simulink model "ctrl_custom"  (R2016b)
settings: Solver=ode4  StartTime=0.0  StopTime=500  FixedStep=0.01  RelTol=1e-3  EnableMultiTasking=on
libraries: simulink x2
(part 2 of 2)

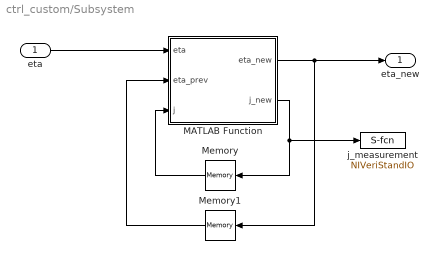
== system ctrl_custom/Subsystem ==
  eta : Inport
  MATLAB Function : MATLAB Function  TreatAsAtomicUnit=on
  Memory : Memory
  Memory1 : Memory  X0=[0;0;0]
  "j_measurement " : S-Function  Priority=1  FunctionName=NIVeriStandIO  Parameters=width dtype portnum stime stype btype  SFunctionDeploymentMode=off  EnableBusSupport=off  mask(NI VeriStand Outport){portnum=1, width=-1, stime=-1, dtype=auto, stype=auto, btype=0}
      mask prompts: portnum "Port number:"; width "Port dimensions (-1 for dynamically sized):"; stime "Sample time (-1 for inherited):"; dtype "Data type:"; stype "Signal type:"; btype "Block type:"
      mask help: Use this outport on any level of nested subsystems to allow NI VeriStand software to map signals to it.
      mask init:
      | NIVeriStandIO_init;
      settings: CopyFcn=NIVeriStand_MDL_functions('', 'IO_copy');  DeleteFcn=NIVeriStand_MDL_functions('', 'IO_delete');  MoveFcn=set_param(gcb, 'Mask', 'on');
      mask Callback portnum: NIVeriStand_MDL_functions('', 'IO_setportnum');
      mask TypeOptions dtype: auto | double | single | int8 | uint8 | int16 | uint16 | int32 | uint32 | boolean
      mask Callback dtype: NIVeriStand_MDL_functions('', 'IO_booleansignal');
      mask TypeOptions stype: auto | real | complex
      mask Display:
      | patch([-x x], [-y y], [.90980 .81960 .32156]);
      | plot([xrad -x x xrad], [yrad -y y yrad]);
      | fprintf('NI Out%d', portnum);
  eta_new : Outport
  wires:
  MATLAB Function/1(eta_new) -> Memory1/1, eta_new/1
  eta/1 -> MATLAB Function/1(eta)
  MATLAB Function/2(j_new) -> "j_measurement "/1, Memory/1
  Memory/1 -> MATLAB Function/3(j)
  Memory1/1 -> MATLAB Function/2(eta_prev)

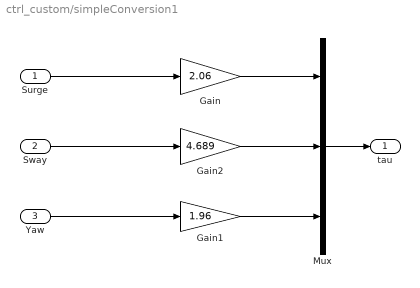
== system ctrl_custom/simpleConversion1 ==
  Surge : Inport
  Sway : Inport  Port=2
  Yaw : Inport  Port=3
  Gain : Gain  Gain=2.06
  Gain1 : Gain  Gain=1.96
  Gain2 : Gain  Gain=4.689
  Mux : Mux  Inputs=3
  "tau " : Outport
  wires:
  Yaw/1 -> Gain1/1
  Gain/1 -> Mux/1
  Mux/1 -> "tau "/1
  Surge/1 -> Gain/1
  Gain1/1 -> Mux/3
  Sway/1 -> Gain2/1
  Gain2/1 -> Mux/2

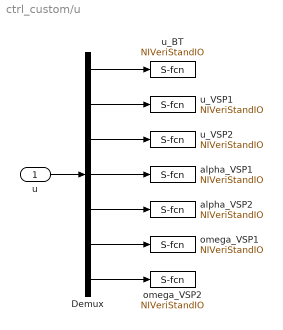
== system ctrl_custom/u ==
  u : Inport
  Demux : Demux  Outputs=7
  alpha_VSP1 : S-Function  Priority=4  FunctionName=NIVeriStandIO  Parameters=width dtype portnum stime stype btype  SFunctionDeploymentMode=off  EnableBusSupport=off  mask(NI VeriStand Outport){portnum=4, width=-1, stime=-1, dtype=auto, stype=auto, btype=0}
      mask prompts: portnum "Port number:"; width "Port dimensions (-1 for dynamically sized):"; stime "Sample time (-1 for inherited):"; dtype "Data type:"; stype "Signal type:"; btype "Block type:"
      mask help: Use this outport on any level of nested subsystems to allow NI VeriStand software to map signals to it.
      mask init:
      | NIVeriStandIO_init;
      settings: CopyFcn=NIVeriStand_MDL_functions('', 'IO_copy');  DeleteFcn=NIVeriStand_MDL_functions('', 'IO_delete');  MoveFcn=set_param(gcb, 'Mask', 'on');
      mask Callback portnum: NIVeriStand_MDL_functions('', 'IO_setportnum');
      mask TypeOptions dtype: auto | double | single | int8 | uint8 | int16 | uint16 | int32 | uint32 | boolean
      mask Callback dtype: NIVeriStand_MDL_functions('', 'IO_booleansignal');
      mask TypeOptions stype: auto | real | complex
      mask Display:
      | patch([-x x], [-y y], [.90980 .81960 .32156]);
      | plot([xrad -x x xrad], [yrad -y y yrad]);
      | fprintf('NI Out%d', portnum);
  alpha_VSP2 : S-Function  Priority=1  FunctionName=NIVeriStandIO  Parameters=width dtype portnum stime stype btype  SFunctionDeploymentMode=off  EnableBusSupport=off  mask(NI VeriStand Outport){portnum=1, width=-1, stime=-1, dtype=auto, stype=auto, btype=0}
      mask prompts: portnum "Port number:"; width "Port dimensions (-1 for dynamically sized):"; stime "Sample time (-1 for inherited):"; dtype "Data type:"; stype "Signal type:"; btype "Block type:"
      mask help: Use this outport on any level of nested subsystems to allow NI VeriStand software to map signals to it.
      mask init:
      | NIVeriStandIO_init;
      settings: CopyFcn=NIVeriStand_MDL_functions('', 'IO_copy');  DeleteFcn=NIVeriStand_MDL_functions('', 'IO_delete');  MoveFcn=set_param(gcb, 'Mask', 'on');
      mask Callback portnum: NIVeriStand_MDL_functions('', 'IO_setportnum');
      mask TypeOptions dtype: auto | double | single | int8 | uint8 | int16 | uint16 | int32 | uint32 | boolean
      mask Callback dtype: NIVeriStand_MDL_functions('', 'IO_booleansignal');
      mask TypeOptions stype: auto | real | complex
      mask Display:
      | patch([-x x], [-y y], [.90980 .81960 .32156]);
      | plot([xrad -x x xrad], [yrad -y y yrad]);
      | fprintf('NI Out%d', portnum);
  omega_VSP1 : S-Function  Priority=2  FunctionName=NIVeriStandIO  Parameters=width dtype portnum stime stype btype  SFunctionDeploymentMode=off  EnableBusSupport=off  mask(NI VeriStand Outport){portnum=2, width=-1, stime=-1, dtype=auto, stype=auto, btype=0}
      mask prompts: portnum "Port number:"; width "Port dimensions (-1 for dynamically sized):"; stime "Sample time (-1 for inherited):"; dtype "Data type:"; stype "Signal type:"; btype "Block type:"
      mask help: Use this outport on any level of nested subsystems to allow NI VeriStand software to map signals to it.
      mask init:
      | NIVeriStandIO_init;
      settings: CopyFcn=NIVeriStand_MDL_functions('', 'IO_copy');  DeleteFcn=NIVeriStand_MDL_functions('', 'IO_delete');  MoveFcn=set_param(gcb, 'Mask', 'on');
      mask Callback portnum: NIVeriStand_MDL_functions('', 'IO_setportnum');
      mask TypeOptions dtype: auto | double | single | int8 | uint8 | int16 | uint16 | int32 | uint32 | boolean
      mask Callback dtype: NIVeriStand_MDL_functions('', 'IO_booleansignal');
      mask TypeOptions stype: auto | real | complex
      mask Display:
      | patch([-x x], [-y y], [.90980 .81960 .32156]);
      | plot([xrad -x x xrad], [yrad -y y yrad]);
      | fprintf('NI Out%d', portnum);
  omega_VSP2 : S-Function  Priority=3  FunctionName=NIVeriStandIO  Parameters=width dtype portnum stime stype btype  SFunctionDeploymentMode=off  EnableBusSupport=off  mask(NI VeriStand Outport){portnum=3, width=-1, stime=-1, dtype=auto, stype=auto, btype=0}
      mask prompts: portnum "Port number:"; width "Port dimensions (-1 for dynamically sized):"; stime "Sample time (-1 for inherited):"; dtype "Data type:"; stype "Signal type:"; btype "Block type:"
      mask help: Use this outport on any level of nested subsystems to allow NI VeriStand software to map signals to it.
      mask init:
      | NIVeriStandIO_init;
      settings: CopyFcn=NIVeriStand_MDL_functions('', 'IO_copy');  DeleteFcn=NIVeriStand_MDL_functions('', 'IO_delete');  MoveFcn=set_param(gcb, 'Mask', 'on');
      mask Callback portnum: NIVeriStand_MDL_functions('', 'IO_setportnum');
      mask TypeOptions dtype: auto | double | single | int8 | uint8 | int16 | uint16 | int32 | uint32 | boolean
      mask Callback dtype: NIVeriStand_MDL_functions('', 'IO_booleansignal');
      mask TypeOptions stype: auto | real | complex
      mask Display:
      | patch([-x x], [-y y], [.90980 .81960 .32156]);
      | plot([xrad -x x xrad], [yrad -y y yrad]);
      | fprintf('NI Out%d', portnum);
  u_BT : S-Function  Priority=5  FunctionName=NIVeriStandIO  Parameters=width dtype portnum stime stype btype  SFunctionDeploymentMode=off  EnableBusSupport=off  mask(NI VeriStand Outport){portnum=5, width=-1, stime=-1, dtype=auto, stype=auto, btype=0}
      mask prompts: portnum "Port number:"; width "Port dimensions (-1 for dynamically sized):"; stime "Sample time (-1 for inherited):"; dtype "Data type:"; stype "Signal type:"; btype "Block type:"
      mask help: Use this outport on any level of nested subsystems to allow NI VeriStand software to map signals to it.
      mask init:
      | NIVeriStandIO_init;
      settings: CopyFcn=NIVeriStand_MDL_functions('', 'IO_copy');  DeleteFcn=NIVeriStand_MDL_functions('', 'IO_delete');  MoveFcn=set_param(gcb, 'Mask', 'on');
      mask Callback portnum: NIVeriStand_MDL_functions('', 'IO_setportnum');
      mask TypeOptions dtype: auto | double | single | int8 | uint8 | int16 | uint16 | int32 | uint32 | boolean
      mask Callback dtype: NIVeriStand_MDL_functions('', 'IO_booleansignal');
      mask TypeOptions stype: auto | real | complex
      mask Display:
      | patch([-x x], [-y y], [.90980 .81960 .32156]);
      | plot([xrad -x x xrad], [yrad -y y yrad]);
      | fprintf('NI Out%d', portnum);
  u_VSP1 : S-Function  Priority=6  FunctionName=NIVeriStandIO  Parameters=width dtype portnum stime stype btype  SFunctionDeploymentMode=off  EnableBusSupport=off  mask(NI VeriStand Outport){portnum=6, width=-1, stime=-1, dtype=auto, stype=auto, btype=0}
      mask prompts: portnum "Port number:"; width "Port dimensions (-1 for dynamically sized):"; stime "Sample time (-1 for inherited):"; dtype "Data type:"; stype "Signal type:"; btype "Block type:"
      mask help: Use this outport on any level of nested subsystems to allow NI VeriStand software to map signals to it.
      mask init:
      | NIVeriStandIO_init;
      settings: CopyFcn=NIVeriStand_MDL_functions('', 'IO_copy');  DeleteFcn=NIVeriStand_MDL_functions('', 'IO_delete');  MoveFcn=set_param(gcb, 'Mask', 'on');
      mask Callback portnum: NIVeriStand_MDL_functions('', 'IO_setportnum');
      mask TypeOptions dtype: auto | double | single | int8 | uint8 | int16 | uint16 | int32 | uint32 | boolean
      mask Callback dtype: NIVeriStand_MDL_functions('', 'IO_booleansignal');
      mask TypeOptions stype: auto | real | complex
      mask Display:
      | patch([-x x], [-y y], [.90980 .81960 .32156]);
      | plot([xrad -x x xrad], [yrad -y y yrad]);
      | fprintf('NI Out%d', portnum);
  u_VSP2 : S-Function  Priority=7  FunctionName=NIVeriStandIO  Parameters=width dtype portnum stime stype btype  SFunctionDeploymentMode=off  EnableBusSupport=off  mask(NI VeriStand Outport){portnum=7, width=-1, stime=-1, dtype=auto, stype=auto, btype=0}
      mask prompts: portnum "Port number:"; width "Port dimensions (-1 for dynamically sized):"; stime "Sample time (-1 for inherited):"; dtype "Data type:"; stype "Signal type:"; btype "Block type:"
      mask help: Use this outport on any level of nested subsystems to allow NI VeriStand software to map signals to it.
      mask init:
      | NIVeriStandIO_init;
      settings: CopyFcn=NIVeriStand_MDL_functions('', 'IO_copy');  DeleteFcn=NIVeriStand_MDL_functions('', 'IO_delete');  MoveFcn=set_param(gcb, 'Mask', 'on');
      mask Callback portnum: NIVeriStand_MDL_functions('', 'IO_setportnum');
      mask TypeOptions dtype: auto | double | single | int8 | uint8 | int16 | uint16 | int32 | uint32 | boolean
      mask Callback dtype: NIVeriStand_MDL_functions('', 'IO_booleansignal');
      mask TypeOptions stype: auto | real | complex
      mask Display:
      | patch([-x x], [-y y], [.90980 .81960 .32156]);
      | plot([xrad -x x xrad], [yrad -y y yrad]);
      | fprintf('NI Out%d', portnum);
  wires:
  u/1 -> Demux/1
  Demux/1 -> u_BT/1
  Demux/2 -> u_VSP1/1
  Demux/3 -> u_VSP2/1
  Demux/4 -> alpha_VSP1/1
  Demux/5 -> alpha_VSP2/1
  Demux/6 -> omega_VSP1/1
  Demux/7 -> omega_VSP2/1

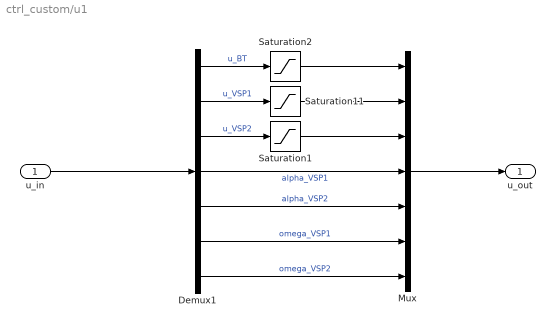
== system ctrl_custom/u1 ==
  u_in : Inport
  Demux1 : Demux  Outputs=7
  Mux : Mux  Inputs=7
  Saturation1 : Saturate  UpperLimit=1  LowerLimit=0
  Saturation11 : Saturate  UpperLimit=1  LowerLimit=0
  Saturation2 : Saturate  UpperLimit=1  LowerLimit=-1
  u_out : Outport
  wires:
  Saturation1/1 -> Mux/3
  Saturation11/1 -> Mux/2
  Mux/1 -> u_out/1
  Demux1/7 -> Mux/7  "omega_VSP2"
  Demux1/6 -> Mux/6  "omega_VSP1"
  Demux1/5 -> Mux/5  "alpha_VSP2"
  Demux1/4 -> Mux/4  "alpha_VSP1"
  Demux1/3 -> Saturation1/1  "u_VSP2"
  Demux1/2 -> Saturation11/1  "u_VSP1"
  Demux1/1 -> Saturation2/1  "u_BT"
  u_in/1 -> Demux1/1
  Saturation2/1 -> Mux/1

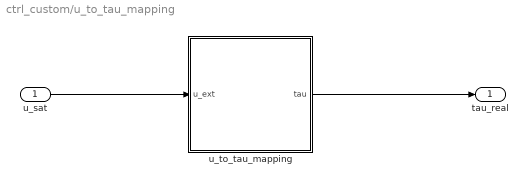
== system ctrl_custom/u_to_tau_mapping ==
  u_sat : Inport
  u_to_tau_mapping : MATLAB Function  TreatAsAtomicUnit=on
  tau_real : Outport
  wires:
  u_sat/1 -> u_to_tau_mapping/1(u_ext)
  u_to_tau_mapping/1(tau) -> tau_real/1

== matlab function ctrl_custom/Control law/MATLAB Function ==
  data: s_reset output; eta_0_new output; eta input; switch_signal_new output; switch_signal input; eta_0 input; switch_signal_prev input
function [s_reset,eta_0_new,switch_signal_new] = control_switch(eta,switch_signal,eta_0,switch_signal_prev)

if switch_signal ~= 0 && switch_signal_prev == 0
    eta_0_new = eta;
    s_reset = 1;
else
    s_reset = 0;
    eta_0_new = eta_0;    
end

switch_signal_new = switch_signal;

== matlab function ctrl_custom/dead_reckoning ==
  data: eta input; bollebutton input; status output; last input; last output; last2 output; last3 output; last2 input; last3 input
function [status, last, last2, last3] = dead_reckoning(eta, bollebutton, last, last2, last3)

if (eta(1) == last(1) && eta(2) == last(2) && eta(3) == last(3) && ...
        eta(1) == last2(1) && eta(2) == last2(2) && eta(3) == last2(3) ...
       && eta(1) == last3(1) && eta(2) == last3(2) && eta(3) == last3(3))
    status = 0;
else
    status = 1;
end

if bollebutton == 1
    status = 0;
end
   
last3 = last2;
last2 = last;
last = eta;

== matlab function ctrl_custom/u_to_tau_mapping/u_to_tau_mapping ==
  data: u_ext input; tau output
function tau = fcn(u_ext)

%% Thruster configuration
Lx_vsp = 0.4574;
Ly_vsp = 0.055;
Lx_bt = 0.3875;

Lx_vsp_1 = -Lx_vsp;
Ly_vsp_1 = -Ly_vsp;
Lx_vsp_2 = -Lx_vsp;
Ly_vsp_2 = Ly_vsp;

k_1 = 1.03;
k_2 = 1.03;
k_3 = 2.629;

K = diag([k_3 k_1 k_2]);

u = u_ext(1:3);

%% Mapping
alpha_vsp1 = u_ext(4);
alpha_vsp2 = u_ext(5);

B = [0          cos(alpha_vsp1)         cos(alpha_vsp2);
     1          sin(alpha_vsp1)         sin(alpha_vsp2);
     Lx_bt       Lx_vsp_1*sin(alpha_vsp1)-Ly_vsp_1*cos(alpha_vsp1)   Lx_vsp_2*sin(alpha_vsp2)-Ly_vsp_2*cos(alpha_vsp2)];
    
tau = B*K*u;
end

== matlab function ctrl_custom/Control law/Control law ==
  data: path input; mu input; U_ref input; rx input; ry input; Kp input; Kd input; s_reset input; eta_0 input; switch_signal input; eta_hat input; nu_hat input; D input; C input; s input; j_path input; tau_cmd output; pd output; s_dot output; j_path_curr output; pd_prev input; pd_curr output
function [tau_cmd, pd, s_dot, j_path_curr, pd_curr] ...
    = control_law(path,mu,U_ref,rx,ry,Kp,Kd,...
    s_reset, eta_0, switch_signal, eta_hat, nu_hat, D, C, s, ...
    j_path, pd_prev)
%% Path parameters

%path = 'ellipsoidal'; % "linear" or "ellipsoidal"

% rx  = 1.5;    % Ellipsoidal x-radius
% ry  = 1;    % Ellipsoidal y-radius

%% Control law parameters

% mu = 0.01;
% U_ref = 0.2;

%% Starting position conditions

p_0   = [   eta_0(1);
            eta_0(2)];
        
p_1   = [   p_0(1) + cos(eta_0(3));
            p_0(2) + sin(eta_0(3))];

p_c   = [   p_0(1) - rx;
            p_0(2)];

% Starting point round counter
rem = mod(eta_0(3,1), 2*pi);
j_pos_0 = (eta_0(3,1) - rem) / (2*pi);

if rem >= pi
   j_pos_0 = j_pos_0 + 1;
end

% Setting pd_prev within the 
if s_reset == 1
    pd_prev = [0, 0, 2*pi*j_pos_0]';
    j_path = 0;
end

%% Rotation and rotation speed matrices

Rot_mat = [cos(eta_hat(3))  -sin(eta_hat(3))    0;
           sin(eta_hat(3))  cos(eta_hat(3))     0;
           0                0                   1];

S_mat = [0          -nu_hat(3)  0;
         nu_hat(3)  0           0;
         0          0           0];

%% Path parameterization

if path == 0    
    pd      =   [   p_0(1) + (p_1(1)-p_0(1))*s;
                    p_0(2) + (p_1(2)-p_0(2))*s;
                    atan2(p_1(2)-p_0(2),p_1(1)-p_0(1))]; 
    pd_s    =   [   p_1(1)-p_0(1);
                    p_1(2)-p_0(2);
                    0];
    pd_ss   =   [   0;
                    0;
                    0];
elseif path == 1
    pd      =   [   p_c(1) + rx*cos(2*pi*s);
                    p_c(2) + ry*sin(2*pi*s);
                    atan2(2*pi*ry*cos(2*pi*s),-2*pi*rx*sin(2*pi*s))];
    pd_s    =   [   -2*pi*rx*sin(2*pi*s);
                    2*pi*ry*cos(2*pi*s);
                    (2*pi*rx*ry) ...
                    / (rx^2*sin(2*pi*s)^2+ry^2*cos(2*pi*s)^2)];
    pd_ss =     [   -4*pi^2*rx*cos(2*pi*s);
                    -4*pi^2*ry*sin(2*pi*s);
                    -(8*pi^2*rx*ry*sin(2*pi*s)*cos(2*pi*s)*(rx^2-ry^2)) ...
                    / ((rx^2*sin(2*pi*s)^2)+(ry^2*cos(2*pi*s)^2)^2)];
else
    pd = [0 0 0]';
    pd_s = [0 0 0]';
    pd_ss = [0 0 0]';
end

%% Calculate path vectors

% pd      = [ p_x;
%             p_y;
%             atan2(p_y_s, p_x_s)];
% pd_s    = [ p_x_s;
%             p_y_s;
%             (p_x_s*p_y_ss - p_y_s*p_x_ss) / (p_x_ss + p_y_ss)];
% pd_ss   = [ p_x_ss;
%             p_y_ss;
%             (p_x_s*p_y_sss - p_y_s*p_x_sss) / ((p_x_s)^2 + (p_y_s)^2) ...
%             - 2 * (p_x_s*p_y_ss - p_y_s*p_x_ss) ...
%             * (p_x_s*p_x_ss + p_y_s*p_y_ss) / ((p_x_s)^2 + (p_y_s)^2)^2];

%% Trajectory round counting

% Round counter for the trajectory
atan2_diff = pd(3,1) - (pd_prev(3,1) - 2*pi*(j_pos_0 + j_path));

if atan2_diff < -pi
    j_path = j_path + 1;
elseif atan2_diff > pi
    j_path = j_path - 1;
end

%% Calculate trajectory heading

pd(3,1) = 2*pi*(j_pos_0 + j_path) + pd(3,1);

%% Update laws

Us    = U_ref / norm(pd_s);

z1 = Rot_mat'*(eta_hat - pd);
V_s   = -(eta_hat-pd)'*pd_s;
omega = mu*V_s / norm(pd_s);


if switch_signal~=0
    s_dot = (Us - omega);
else
    s_dot = 0;
end

Us_s  = (-U_ref*((pd_s(1)*pd_ss(1))+(pd_s(2)*pd_ss(2)))) ...
        / (pd_s(1)^2 + pd_s(2)^2)^(3/2);
Us_dot = Us_s * s_dot;


alpha1 = -Kp*z1 + pd_s*Us;

%% Control law

% Include bias and coriolis matrix?
M = [16.11 0 0; 0 24.11 0.53; 0 0.53 2.76];

alpha1_dot = ...
    Kp*(S_mat*z1 - nu_hat) ...
    - S_mat*Rot_mat'*pd_s*Us ...
    + Rot_mat'*pd_s*Us_dot ...
    + (Kp*Rot_mat'*pd_s + Rot_mat'*(pd_ss*Us + pd_s*Us_s))*s_dot;

z2 = nu_hat - alpha1;

%% Switch logics

if switch_signal~=0
    tau_cmd = -z1 + D*nu_hat + C*nu_hat + M*alpha1_dot - Kd*z2;
else
    tau_cmd = zeros(3,1);
end

%% Assign variables for memory blocks

j_path_curr = j_path;
pd_curr = pd;
pd_s_curr = pd_s;
pd_ss_curr = pd_ss;

end

== matlab function ctrl_custom/Rectangular coordinate thrust allocation/MATLAB Function ==
  data: tau input; u_ext output
function u_ext = fcn(tau)

%%
%Initialize extended thrust allocation matrix
L_xvsp = 0.4574;
L_yvsp = 0.055;
L_bt = 0.3875;

L_xvsp_1 = -L_xvsp;
L_yvsp_1 = -L_yvsp;
L_xvsp_2 = -L_xvsp;
L_yvsp_2 = L_yvsp;

B_ext = [1         0        1         0        0;
     0         1        0         1        1;
     -L_yvsp_1 L_xvsp_1 -L_yvsp_2 L_xvsp_2 L_bt];
 
B_ext_inv = pinv(B_ext);

%Extended force vector
f = B_ext_inv*tau;

%%
%Calculate angles and control input
alpha_1 = atan2(f(2), f(1));
alpha_2 = atan2(f(4), f(3));

alpha = [alpha_1; alpha_2];

k_1 = 2.629;
k_2 = 1.03;
k_3 = 1.03;

u_1 = (1/k_2)*sqrt(f(1)^2 + f(2)^2);
u_2 = (1/k_3)*sqrt(f(3)^2 + f(4)^2);
u_3 = f(5)/k_1;

u = [u_1; u_2; u_3];

u_ext = [u; alpha];

== matlab function ctrl_custom/Subsystem/MATLAB Function ==
  data: eta input; eta_new output; eta_prev input; j input; j_new output
function [eta_new, j_new] = fcn(eta, eta_prev, j)

eta = diag([1/1000 1/1000 pi/180])*eta;

if (eta(3,1) - (eta_prev(3,1)-2*pi*j)) < -pi
    j_new = j + 1;
elseif (eta(3,1) - (eta_prev(3,1)-2*pi*j)) > pi
    j_new = j - 1;
else
     j_new = j;
end

eta_new = eta;

eta_new(3,1) = 2*pi*j_new + eta(3,1);

== matlab function ctrl_custom/Observer/MATLAB Function ==
  data: u input; D output
function D = fcn(u)

d11 = 0.6555;   %% - 0.3545*sqrt(u(1)^2) + 3.787*u(1)^2;
d22 = 1.33;     %% + 2.776*sqrt(u(2)^2) + 64.91*u(2)^2 + 0.805*sqrt(u(2)^2);
d23 = 7.25;     %% + 0.845*sqrt(u(2)^2) +3.45*sqrt(u(3)^2);
d32 = 0;        %%0.2088*sqrt(u(2)^2) - 0.130*sqrt(u(3)^2);
d33 = 1.9;      % - 0.080*sqrt(u(3)^2) + 0.75*sqrt(u(3)^2);

D = [d11    0       0;
     0      d22     d23;
     0      d32     d33];

== matlab function ctrl_custom/Observer/rotation matrix ==
  data: psi input; y output
function y = rotation_matrix(psi)

y = [cos(psi) -sin(psi) 0;
    sin(psi) cos(psi) 0;
    0 0 1];
 end

== matlab function ctrl_custom/Observer/Inverse ==
  data: u input; y output
function y = fcn(u)


y = inv(u);

== matlab function ctrl_custom/Observer/Transpose ==
  data: u input; y output
function y = fcn(u)


y = u.';

== matlab function ctrl_custom/Control law/Damping and coriolis ==
  data: D output; nu_hat input; C output
function [D,C] = damp_cori_calculator(nu_hat)
%% MATRICES
m    = 14.11;   I_z  =  1.7600;   x_g = 0.0375;       % x_g  =  0.0460; % Table B.1

%% Added mass
X_ud  =     -2.0;											% Table B.1
					Y_vd =     -10.0;	N_vd =    -0.0;		% Table B.1
					Y_rd =      -0.0;	N_rd =    -1.0;		% Table B.1

%% Total mass matrix
m_11 = m-X_ud;
m_22 = m-Y_vd;
m_23 = m*x_g-Y_rd;
m_32 = m*x_g-N_vd;
m_33 = I_z-N_rd;

M    = [m_11 0    0
        0    m_22 m_23
        0    m_32 m_33];
	
%% Damping coefficients
% Comments at the end of the lines indicate the old values used.
X_u		= -0.6555;		X_v		= 0;
X_uu 	= 0.3545;		X_vv	= -2.443;
X_uuu 	= -3.787;		X_vvv	= 0;

						Y_v		= -1.33; 			Y_r		= -7.250; % Y_r
						Y_vv	= -2.776;			Y_rr	= -3.450; % Y_rr
						Y_vvv	= -64.91;			Y_rrr	= 0;
						
						Y_rv	= -0.805;			Y_vr	= -0.845; % Y_rv, Y_vr

						N_v		= 0;				N_r		= -1.900; % N_r
						N_vv	= -0.2088;			N_rr	= -0.750; % N_rr
						N_vvv	= 0;				N_rrr	= 0;
						
						N_rv	= 0.130;			N_vr	= 0.080; % N_rv, N_vr

%% Correolis matrix
c_13 = -(m-Y_vd)*nu_hat(2)-(m*x_g-Y_rd)*nu_hat(3);
c_23 = (m-X_ud)*nu_hat(1);
C    = [0     0     c_13
        0     0     c_23
        -c_13 -c_23 0   ];

%% Assembly of the damping matrix
d_11 = -X_u - X_uu*abs(nu_hat(1)) - X_uuu*nu_hat(1)^2;
d_22 = -Y_v - Y_vv*abs(nu_hat(2)) - Y_vvv*nu_hat(2)^2 - Y_rv*abs(nu_hat(3));
d_33 = -N_r - N_rr*abs(nu_hat(3)) - N_rrr*nu_hat(3)^2 - N_vr*abs(nu_hat(2));

d_23 = -Y_r - Y_rr*abs(nu_hat(3)) - Y_rrr*nu_hat(3)^2 - Y_vr*abs(nu_hat(2));
d_32 = -N_v - N_vv*abs(nu_hat(2)) - N_vvv*nu_hat(2)^2 - N_rv*abs(nu_hat(3));

D    = [d_11 0 0
        0    d_22 d_23
        0    d_32 d_33];
